simulink model "S2_Boost_model_ideal"  (R2022a)
settings: Solver=VariableStepAuto  StartTime=0.0  StopTime=spec.sim_time  FixedStep=1e-8  MaxStep=1e-7  RelTol=1e-1
undefined symbols (not defined in the file): ideal, spec
libraries: fl_lib x16, nesl_utility x12, spsMeanLib x5, spsRMSLib x3, ee_lib x1, spsPWMGeneratorDCDCLib x1
settings Model: Creator=delta  LastModifiedBy=delta
settings SolverCC: MaxConsecutiveZCs=100  ZeroCrossAlgorithm=Adaptive
settings DebuggingCC: IgnoredZcDiagnostic=none  UnconnectedInputMsg=warning  UnconnectedOutputMsg=warning  UnconnectedLineMsg=warning
settings RTWCC: DLArmComputeVersion=19.05

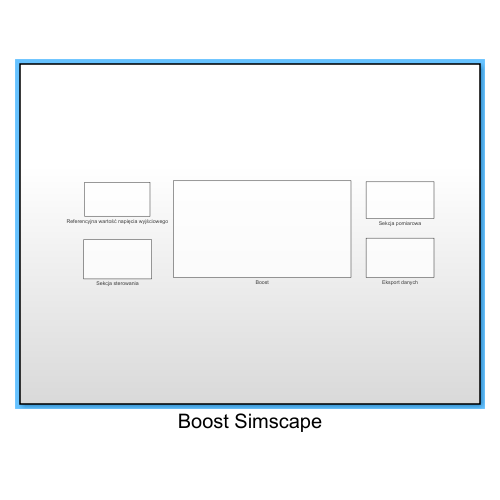
[thumbnail: Simulink's stored preview of the top-level diagram]
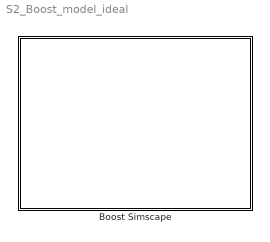
== system S2_Boost_model_ideal ==
  Boost Simscape : Subsystem

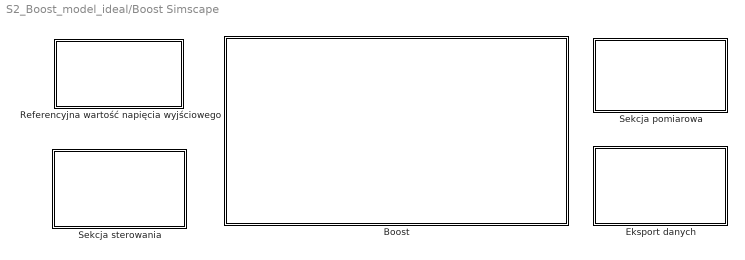
== system S2_Boost_model_ideal/Boost Simscape ==
  Boost : Subsystem
  Eksport danych : Subsystem
  Referencyjna wartość napięcia wyjściowego : Subsystem
  Sekcja pomiarowa : Subsystem
  Sekcja sterowania : Subsystem

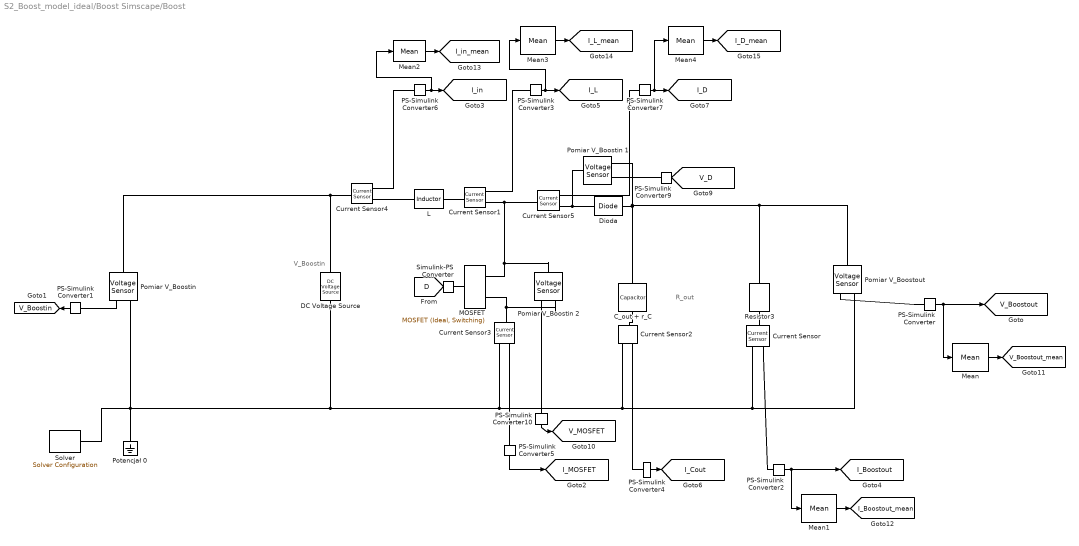
== system S2_Boost_model_ideal/Boost Simscape/Boost ==
  note: V_Boostin
  note: R_out
  C_out + r_C : fl_lib/Electrical/Electrical Elements/Capacitor  c="ideal.Cout.calc.C_out   F"  r=0 Ohm  g=0 1/Ohm  i_specify=off  i_priority=None  i=0 A  i_nominal_specify=off  i_nominal_unit=A  i_nominal_value=1  v_specify=off  v_priority=None  v=0 V  v_nominal_specify=off  v_nominal_unit=V  v_nominal_value=1  vc_specify=off  vc_priority=High  vc=0 V  vc_nominal_specify=off  vc_nominal_unit=V  vc_nominal_value=1
      settings: SourceProductBaseCode=PW,SS,VE
  Current Sensor{,1..5} (6 alike) : fl_lib/Electrical/Electrical Sensors/Current Sensor
      settings: SourceProductBaseCode=PW,SS,VE
  DC Voltage Source : fl_lib/Electrical/Electrical Sources/DC Voltage Source  v0=spec.V_in V
      settings: SourceProductBaseCode=PW,SS,VE
  Dioda : fl_lib/Electrical/Electrical Elements/Diode  Vf=1e-9 V  Ron=1e-9 Ohm  Goff=1e-9 1/Ohm  i_specify=off  i_priority=None  i=0 A  i_nominal_specify=off  i_nominal_unit=A  i_nominal_value=1  v_specify=off  v_priority=None  v=0 V  v_nominal_specify=off  v_nominal_unit=V  v_nominal_value=1
      settings: SourceProductBaseCode=PW,SS,VE
  L : fl_lib/Electrical/Electrical Elements/Inductor  l=ideal.L.calc.L_min H  r=0 Ohm  g=0 1/Ohm  i_specify=off  i_priority=None  i=0 A  i_nominal_specify=off  i_nominal_unit=A  i_nominal_value=1  v_specify=off  v_priority=None  v=0 V  v_nominal_specify=off  v_nominal_unit=V  v_nominal_value=1  i_L_specify=off  i_L_priority=High  i_L=0 A  i_L_nominal_specify=off  i_L_nominal_unit=A  i_L_nominal_value=1
      settings: SourceProductBaseCode=PW,SS,VE
  "MOSFET " : ee_lib/Semiconductors & Converters/MOSFET (Ideal, Switching)  Rds=1e-9 Ohm  Goff=1e-6 1/Ohm  Vth=0 V  diode_param=1  diode_Vf=0.8 V  diode_Ron=0.001 Ohm  diode_Goff=1e-5 1/Ohm  diode_C=50e-9 F  diode_iRM=-235 A  diode_iF=300 A  diode_idot=-50 A/us  diode_trr_param=1  diode_trr_factor=3  diode_trr=15 us  diode_Qrr=1500 s*uA  thermal_loss_option=ee.enum.converters.thermalLossOption.constantvalues  Von_data=[0, 1.1, 1.3, 1.45, 1.75, 2.25, 2.7; 0, 1, 1.15, 1.35, 1.7, 2.35, 3] V  Tj=[298.15, 398.15] K  Iout_data=[0, 10, 50, 100, 200, 400, 600] A  Eon_data=[0, .29, 1.43, 2.86, 5.71, 13.14, 22.86; 0, .57, 2.63, 5.14, 10.29, 20.57, 30.29] * 1e-3 J  Eoff_data=[0, .21, 1.07, 2.14, 4.29, 9.86, 17.14; 0, .43, 1.97, 3.86, 7.71, 15.43, 22.71] * 1e-3 J  Tj_loss=[298.15, 398.15] K  Iout_data_loss=[0, 10, 50, 100, 200, 400, 600] A  Eon_scalar=22.86e-3 J  Eoff_scalar=17.14e-3 J  Voff=300 V  Iout_scalar=600 A  diodeModelType=ee.enum.converters.diodeModelType.pwl  diodeTableType=ee.enum.diode.tableType.IfMat  diode_IfMat=[.07, .12, .19, 1.75, 4.24, 7.32, 11.2; .16, .3, .72, 2.14, 4.02, 6.35, 9.12] A  diode_VfMat=[.9, 1.15, 1.25, 1.5, 1.75, 2.17, 2.6, 2.85; .58, .68, .75, 1.1, 1.38, 1.77, 2.27, 2.7] V  diode_TjVec=[25, 125] degC  diode_VfVec=[.5, .7, .9, 1.3, 1.7, 2.1, 2.5] V  diode_IfVec=[.1, .2, .5, 1, 2, 4, 7, 10] A  diode_Vr=-600 V  diode_Ls=150 nH  diode_Erec=0.03 J  thermal_network_parameterization=ee.enum.thermalNetworkTopology.external  Rth=[.03, .2] K/W  Rth_Cauer=[.03, .1, .2] K/W  Rth_Foster=[.03, .2] K/W  thermal_mass_parameterization=ee.enum.thermalNetwork.timeconstant  thermal_mass=[3, 25] J/K  thermal_mass_Cauer=[3, 10, 25] J/K  thermal_mass_Foster=[33, 50] J/K  thermal_time_constant=[.1, 5] s  thermal_time_constant_Cauer=[.1, 1, 5] s  thermal_time_constant_Foster=[1, 10] s  thermal_mass_initial_temperatures=[25, 25] degC  thermal_mass_initial_temperatures_Cauer=[25, 25, 25] degC  junction_thermal_mass=0.1 J/K  steadyState_Foster=simscape.enum.onoff.on  Tvec_initial_Foster=[25, 25, 25, 25] degC  no_thermal_network=0  junction_temperature_specify=off  junction_temperature_priority=None  junction_temperature=25 degC  junction_temperature_nominal_specify=off  junction_temperature_nominal_unit=degC  junction_temperature_nominal_value=1  vT_specify=off  vT_priority=None  vT=0 V  vT_nominal_specify=off  vT_nominal_unit=V  vT_nominal_value=1  Qj_specify=off  Qj_priority=None  Qj=0 W  Qj_nominal_specify=off  Qj_nominal_unit=W  Qj_nominal_value=1
  Mean{,1..4} (5 alike) : spsMeanLib/Mean  Freq=spec.f_s  Vinit=0  Ts=0
  PS-Simulink Converter{,1..7,9..10} (10 alike) : nesl_utility/PS-Simulink Converter  PhysicalDomain=network_engine_domain  SubClassName=ps_output  LeftPortType=input  RightPortType=output  PseudoPeriodic=off  Frequencies=[]  VectorFormat=1-D array  Unit=inherit  AffineConversion=off
      settings: SourceProductBaseCode=SS,PW,VE
  "Pomiar V_Boostin " : fl_lib/Electrical/Electrical Sensors/Voltage Sensor
      settings: SourceProductBaseCode=PW,SS,VE
  Pomiar V_Boostin 1 : fl_lib/Electrical/Electrical Sensors/Voltage Sensor
      settings: SourceProductBaseCode=PW,SS,VE
  Pomiar V_Boostin 2 : fl_lib/Electrical/Electrical Sensors/Voltage Sensor
      settings: SourceProductBaseCode=PW,SS,VE
  "Pomiar V_Boostout " : fl_lib/Electrical/Electrical Sensors/Voltage Sensor
      settings: SourceProductBaseCode=PW,SS,VE
  Potencjał 0 : fl_lib/Electrical/Electrical Elements/Electrical Reference
      settings: SourceProductBaseCode=PW,SS,VE
  Resistor3 : fl_lib/Electrical/Electrical Elements/Resistor  R=ideal.general.calc.R_out Ohm  i_specify=off  i_priority=None  i=0 A  i_nominal_specify=off  i_nominal_unit=A  i_nominal_value=1  v_specify=off  v_priority=None  v=0 V  v_nominal_specify=off  v_nominal_unit=V  v_nominal_value=1
      settings: SourceProductBaseCode=PW,SS,VE
  Simulink-PS Converter : nesl_utility/Simulink-PS Converter  PhysicalDomain=network_engine_domain  SubClassName=ps_input  LeftPortType=input  RightPortType=output  PseudoPeriodic=off  Frequencies=[]  NoiseDistribution=none  NoiseParameters=[]  Unit=1  AffineConversion=off  FilteringAndDerivatives=provide  SimscapeFilterOrder=1  InputFilterTimeConstant=0.001  UdotUserProvided=0
      settings: SourceProductBaseCode=SS,PW,VE
  "Solver " : nesl_utility/Solver Configuration  PhysicalDomain=network_engine_domain  SubClassName=solver  LeftPortType=input  RightPortType=generic  Tones=[]  Harmonics=[]  SimulateNoise=off  Profile=off  UseLocalSampling=off  EnableSwitchedLinearOptims=on  FrequencyDomain=off  UseCCode=off  RelTol=0.001  AbsTol=1e-06  MinStep=1e-09  ToWorkspace=off  RevertToSquareIcSolve=off  NumHomotopyIterations=100  PhasorMode=off  PhasorModeNumHarmonics=1  IndexReductionMethod=DerivativeReplacement  DoDC=off  ResidualTolerance=1e-07  UseLocalSolver=off  LocalSolverChoice=NE_BACKWARD_EULER_ADVANCER  LocalSolverSampleTime=0.001  DoFixedCost=on  MaxNonlinIter=3  MaxModeIter=2  ComputeImpulses=off  ImpulseIterations=2  LinearAlgebra=auto  LinearAlgebraNumThread=0  EquationFormulation=NE_TIME_EF  DelaysMemoryBudget=1024  AutomaticFiltering=on  FilteringTimeConstant=0.001  PartitionStorageMethod=AS_NEEDED  PartitionMemoryBudget=1024  PartitionMethod=ROBUST
      settings: SourceProductBaseCode=SS,PW,VE
  tag scope: I_Boostout=global, I_Boostout_mean=global, I_Cout=global, I_D=global, I_D_mean=global, I_L=global, I_L_mean=global, I_MOSFET=global, I_in=global, I_in_mean=global, V_Boostin=global, V_Boostout=global, V_Boostout_mean=global, V_D=global, V_MOSFET=global
  wires:
  PS-Simulink Converter/1 -> Mean/1, [V_Boostout]
  PS-Simulink Converter2/1 -> Mean1/1, [I_Boostout]
  [D] -> Simulink-PS Converter/1
  PS-Simulink Converter1/1 -> [V_Boostin]
  PS-Simulink Converter3/1 -> Mean3/1, [I_L]
  PS-Simulink Converter5/1 -> [I_MOSFET]
  PS-Simulink Converter6/1 -> Mean2/1, [I_in]
  PS-Simulink Converter7/1 -> Mean4/1, [I_D]
  PS-Simulink Converter9/1 -> [V_D]
  PS-Simulink Converter10/1 -> [V_MOSFET]
  PS-Simulink Converter4/1 -> [I_Cout]
  Mean/1 -> [V_Boostout_mean]
  Mean1/1 -> [I_Boostout_mean]
  Mean2/1 -> [I_in_mean]
  Mean3/1 -> [I_L_mean]
  Mean4/1 -> [I_D_mean]
  connections:
  "Pomiar V_Boostin "/LConn1 -- DC Voltage Source/LConn1 -- Current Sensor4/LConn1
  Current Sensor/LConn1 -- Resistor3/RConn1
  Current Sensor1/RConn2 -- Pomiar V_Boostin 2/LConn1 -- "MOSFET "/RConn1 -- Current Sensor5/LConn1
  C_out + r_C/RConn1 -- Current Sensor2/LConn1
  PS-Simulink Converter4/LConn1 -- Current Sensor2/RConn1
  Current Sensor/RConn2 -- "Solver "/RConn1 -- Potencjał 0/LConn1 -- "Pomiar V_Boostin "/RConn2 -- DC Voltage Source/RConn1 -- Current Sensor3/RConn2 -- Current Sensor2/RConn2 -- "Pomiar V_Boostout "/RConn2
  C_out + r_C/LConn1 -- Pomiar V_Boostin 1/RConn2 -- "Pomiar V_Boostout "/LConn1 -- Resistor3/LConn1 -- Dioda/RConn1
  Current Sensor/RConn1 -- PS-Simulink Converter2/LConn1
  "MOSFET "/LConn1 -- Simulink-PS Converter/RConn1
  PS-Simulink Converter3/LConn1 -- Current Sensor1/RConn1
  PS-Simulink Converter/LConn1 -- "Pomiar V_Boostout "/RConn1
  Current Sensor1/LConn1 -- L/RConn1
  PS-Simulink Converter1/LConn1 -- "Pomiar V_Boostin "/RConn1
  Current Sensor3/LConn1 -- Pomiar V_Boostin 2/RConn2 -- "MOSFET "/RConn2
  PS-Simulink Converter5/LConn1 -- Current Sensor3/RConn1
  Current Sensor4/RConn2 -- L/LConn1
  Current Sensor4/RConn1 -- PS-Simulink Converter6/LConn1
  Current Sensor5/RConn2 -- Pomiar V_Boostin 1/LConn1 -- Dioda/LConn1
  Current Sensor5/RConn1 -- PS-Simulink Converter7/LConn1
  PS-Simulink Converter9/LConn1 -- Pomiar V_Boostin 1/RConn1
  PS-Simulink Converter10/LConn1 -- Pomiar V_Boostin 2/RConn1

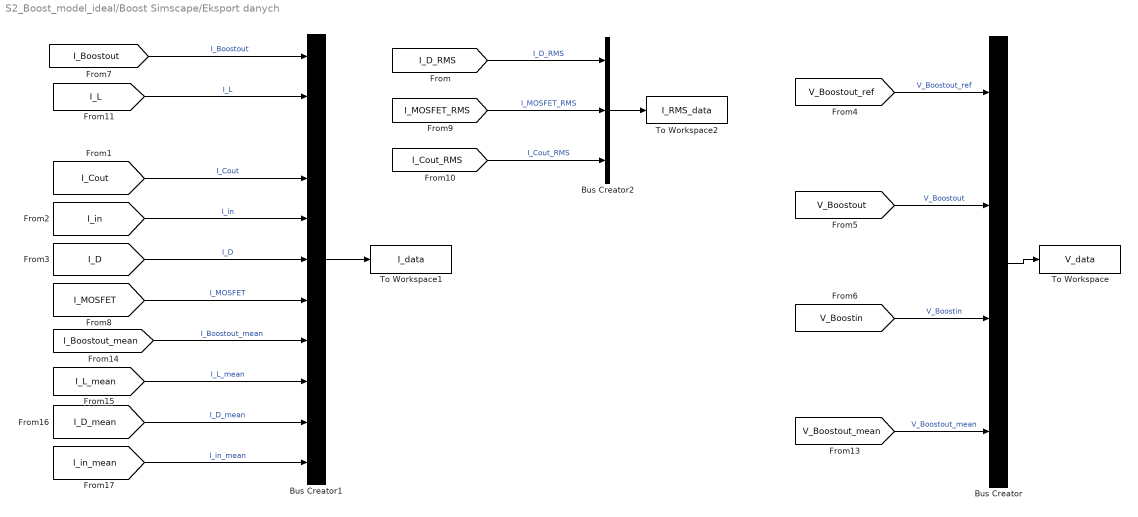
== system S2_Boost_model_ideal/Boost Simscape/Eksport danych ==
  Bus Creator : BusCreator  Inputs=4
  Bus Creator1 : BusCreator  Inputs=11
  Bus Creator2 : BusCreator  Inputs=3
  To Workspace : ToWorkspace  VariableName=V_data  SaveFormat=Timeseries  SampleTime=-1
  To Workspace1 : ToWorkspace  VariableName=I_data  SaveFormat=Timeseries  SampleTime=-1
  To Workspace2 : ToWorkspace  VariableName=I_RMS_data  SaveFormat=Timeseries  SampleTime=-1
  wires:
  [V_Boostin] -> Bus Creator/3  "V_Boostin"
  Bus Creator/1 -> To Workspace/1
  [V_Boostout_ref] -> Bus Creator/1  "V_Boostout_ref"
  [V_Boostout] -> Bus Creator/2  "V_Boostout"
  [I_Boostout] -> Bus Creator1/1  "I_Boostout"
  [I_Cout] -> Bus Creator1/4  "I_Cout"
  [I_L] -> Bus Creator1/2  "I_L"
  [I_in] -> Bus Creator1/5  "I_in"
  [I_D] -> Bus Creator1/6  "I_D"
  [I_MOSFET] -> Bus Creator1/7  "I_MOSFET"
  Bus Creator1/1 -> To Workspace1/1
  [I_D_RMS] -> Bus Creator2/1  "I_D_RMS"
  [I_MOSFET_RMS] -> Bus Creator2/2  "I_MOSFET_RMS"
  Bus Creator2/1 -> To Workspace2/1
  [I_Cout_RMS] -> Bus Creator2/3  "I_Cout_RMS"
  [V_Boostout_mean] -> Bus Creator/4  "V_Boostout_mean"
  [I_Boostout_mean] -> Bus Creator1/8  "I_Boostout_mean"
  [I_L_mean] -> Bus Creator1/9  "I_L_mean"
  [I_D_mean] -> Bus Creator1/10  "I_D_mean"
  [I_in_mean] -> Bus Creator1/11  "I_in_mean"

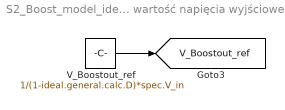
== system S2_Boost_model_ideal/Boost Simscape/Referencyjna wartość napięcia wyjściowego ==
  V_Boostout_ref : Constant  Value=1/(1-ideal.general.calc.D)*spec.V_in
  tag scope: V_Boostout_ref=global
  wires:
  V_Boostout_ref/1 -> [V_Boostout_ref]

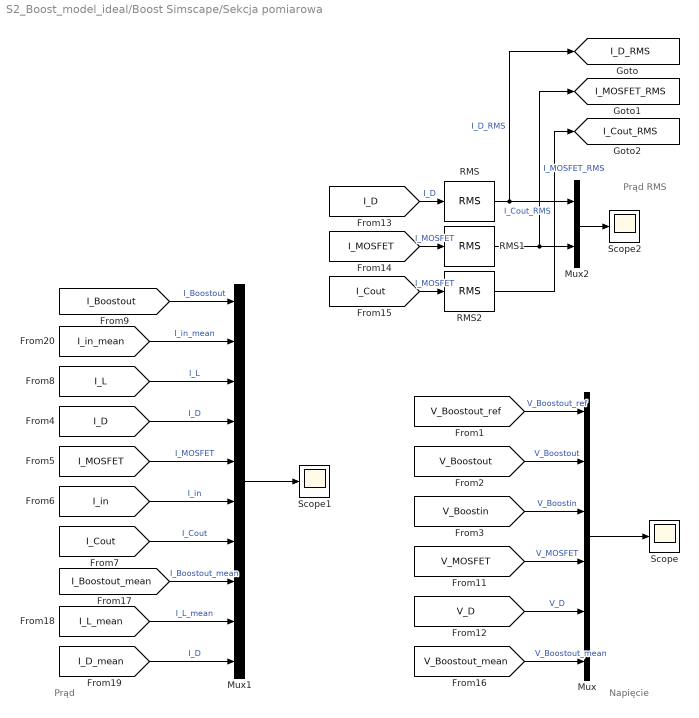
== system S2_Boost_model_ideal/Boost Simscape/Sekcja pomiarowa ==
  note: Napięcie
  note: Prąd
  note: Prąd RMS
  Mux : Mux  Inputs=6
  Mux1 : Mux  Inputs=10
  Mux2 : Mux  Inputs=2
  RMS : spsRMSLib/RMS  TrueRMS=on  Freq=spec.f_s  RMSInit=0  Ts=0
  RMS1 : spsRMSLib/RMS  TrueRMS=on  Freq=spec.f_s  RMSInit=0  Ts=0
  RMS2 : spsRMSLib/RMS  TrueRMS=on  Freq=spec.f_s  RMSInit=0  Ts=0
  Scope : Scope
  Scope1 : Scope
  Scope2 : Scope
  tag scope: I_Cout_RMS=global, I_D_RMS=global, I_MOSFET_RMS=global
  wires:
  [V_Boostout_ref] -> Mux/1  "V_Boostout_ref"
  [I_L] -> Mux1/3  "I_L"
  Mux/1 -> Scope/1
  Mux1/1 -> Scope1/1
  [V_Boostin] -> Mux/3  "V_Boostin"
  [I_Boostout] -> Mux1/1  "I_Boostout"
  [V_Boostout] -> Mux/2  "V_Boostout"
  [I_MOSFET] -> Mux1/5  "I_MOSFET"
  [I_D] -> Mux1/4  "I_D"
  [I_in] -> Mux1/6  "I_in"
  [I_Cout] -> Mux1/7  "I_Cout"
  [V_MOSFET] -> Mux/4  "V_MOSFET"
  [V_D] -> Mux/5  "V_D"
  [I_D] -> RMS/1  "I_D"
  [I_MOSFET] -> RMS1/1  "I_MOSFET"
  RMS/1 -> [I_D_RMS], Mux2/1  "I_D_RMS"
  RMS1/1 -> [I_MOSFET_RMS], Mux2/2  "I_MOSFET_RMS"
  Mux2/1 -> Scope2/1
  [I_Cout] -> RMS2/1  "I_MOSFET"
  RMS2/1 -> [I_Cout_RMS]  "I_Cout_RMS"
  [V_Boostout_mean] -> Mux/6  "V_Boostout_mean"
  [I_Boostout_mean] -> Mux1/8  "I_Boostout_mean"
  [I_L_mean] -> Mux1/9  "I_L_mean"
  [I_D_mean] -> Mux1/10  "I_D"
  [I_in_mean] -> Mux1/2  "I_in_mean"

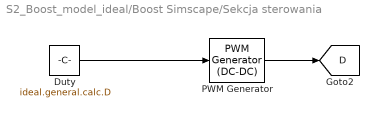
== system S2_Boost_model_ideal/Boost Simscape/Sekcja sterowania ==
  Duty : Constant  Value=ideal.general.calc.D
  "PWM Generator " : spsPWMGeneratorDCDCLib/PWM Generator (DC-DC)  Fsw=spec.f_s  Ts=0
  tag scope: D=global
  wires:
  "PWM Generator "/1 -> [D]
  Duty/1 -> "PWM Generator "/1
